simulink model "three_phase_inverter_reminder"  (R2020b)
settings: Solver=VariableStepAuto  StartTime=0.0  StopTime=0.3  RelTol=1e-3
InitFcn:
  | Tsys = 2e-6;
  | Udc = 380;
  | Tpwm = 1e-4;
  | 
  | Rload = 5
  | Lload = 5e-3
libraries: powerlib x25, simulink x1
settings Model: Creator=messer  LastModifiedBy=messer

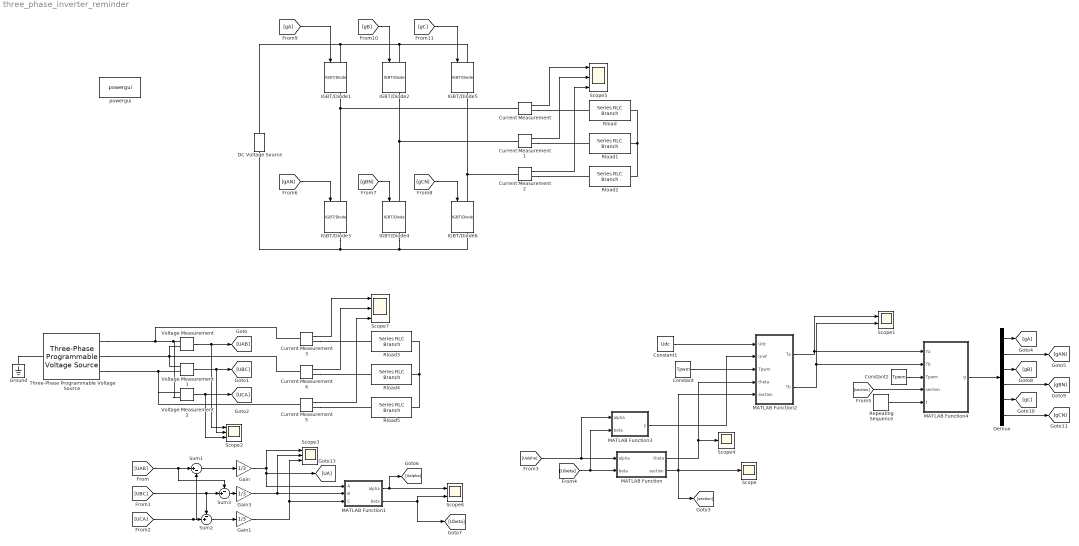
== system three_phase_inverter_reminder ==
  Constant : Constant  Value=Tpwm
  Constant1 : Constant  Value=Udc
  Constant2 : Constant  Value=Tpwm
  Current Measurement{,1..5} (6 alike) : powerlib/Measurements/Current Measurement  PhasorSimulation=off  OutputType=Complex  PSBequivalent=0
  DC Voltage Source : powerlib/Electrical Sources/DC Voltage Source  Amplitude=Udc  Measurements=None
  Demux : Demux  Outputs=6
  Gain : Gain  Gain=1/3
  Gain1 : Gain  Gain=1/3
  Gain3 : Gain  Gain=1/3
  Ground : powerlib/Elements/Ground  LConnTagsString=a
  IGBT/Diode{1..6} (6 alike) : powerlib/Power Electronics/IGBT//Diode  Ron=1e-3  Rs=1e5  Cs=inf  Measurements=on
  MATLAB Function : MATLAB Function  TreatAsAtomicUnit=on
  MATLAB Function1 : MATLAB Function  TreatAsAtomicUnit=on
  MATLAB Function2 : MATLAB Function  TreatAsAtomicUnit=on
  MATLAB Function3 : MATLAB Function  TreatAsAtomicUnit=on
  MATLAB Function4 : MATLAB Function  TreatAsAtomicUnit=on
  Repeating Sequence : simulink/Sources/Repeating Sequence  rep_seq_t=[0 Tpwm]  rep_seq_y=[0 Tpwm]
  Rload{,1..5} (6 alike) : powerlib/Elements/Series RLC Branch  LConnTagsString=__new0  RConnTagsString=__new0  BranchType=RL  Resistance=Rload  Inductance=Lload  SetiL0=off  InitialCurrent=0  Capacitance=1e-6  Setx0=off  InitialVoltage=0  Measurements=None
  Scope : Scope
  Scope1 : Scope  NumInputPorts=2
  Scope{2..3,5,7} (4 alike) : Scope  NumInputPorts=3
  Scope4 : Scope
  Scope6 : Scope  NumInputPorts=2
  Sum1 : Sum  Inputs=|+-
  Sum2 : Sum  Inputs=-+|
  Sum3 : Sum  Inputs=-+|
  Three-Phase Programmable Voltage Source : powerlib/Electrical Sources/Three-Phase Programmable Voltage Source  PositiveSequence="[380/sqrt(2)  0 50]"  VariationEntity=None  VariationType=Table of time-amplitude pairs  VariationTypeAlt=Step  VariationStep=0.5  VariationRate=10  VariationMagnitude=0.3  VariationFrequency=2  VariationTiming=[1 2]  VariationPhaseA=off  Amplitudes=[1 0.8 1.2 1.0]  TimeValues=[0 0.1 0.15 0.2]  HarmonicGeneration=off  HarmonicA=[3 0.2 -25 0]  HarmonicB=[2 0.15 35 2]  Timing="[0.05  3]"  BusType=swing  Pref=0  Qref=0  Qmin=-inf  Qmax=inf
  Voltage Measurement : powerlib/Measurements/Voltage Measurement  PhasorSimulation=off  OutputType=Complex  PSBequivalent=0
  Voltage Measurement1 : powerlib/Measurements/Voltage Measurement  PhasorSimulation=off  OutputType=Complex  PSBequivalent=0
  Voltage Measurement2 : powerlib/Measurements/Voltage Measurement  PhasorSimulation=off  OutputType=Complex  PSBequivalent=0
  powergui : powerlib/powergui  Priority=1  SimulationMode=Discrete  SampleTime=Tsys  frequency=60  Iterations=50  frequencyindice=50  Pbase=100e6  ErrMax=1e-4  UnitsV=kV  UnitsW=MW  buscounter=0  FunctionMessages=off  echomessages=off  EnableUseOfTLC=off  CurrentSourceSwitches=off  DisableSnubberDevices=off  DisableRonSwitches=off  DisableVfSwitches=off  DisplayEquations=off  AutomaticDiscreteSolvers=off  SolverType=Tustin/Backward Euler (TBE)  Interpol=off  ExternalGateDelay=off  methode=off  Ts=100  x0status=blocks  SPID=on  SwTol=0  HookPort=off  NonlinearTolerance=1e-4  nMaxIteration=100  ContinueOnMaxIteration=off  RestoreLinks=warning  ResistiveCurrentMeasurement=off  Frange=[0:2:500]  Ylog=off  Xlog=on  ShowGrid=off  save=off  variable=ZData  structure=0  ZoomFFT=off  StartTime=0.0  cycles=1  DisplayStyle=1  fundamental=60  FreqAxis=off  MaxFrequency=1000  frequencyindicesteady=1  RmsSteady=1  display=off
  wires:
  Voltage Measurement1/1 -> [UBC], Scope2/2
  Voltage Measurement2/1 -> [UCA], Scope2/3
  Voltage Measurement/1 -> Scope2/1, [UAB]
  Sum3/1 -> Gain3/1
  Sum1/1 -> Gain/1
  Gain3/1 -> MATLAB Function1/2(B), Scope3/2
  [UBC] -> Sum2/1, Sum3/2
  MATLAB Function1/1(alpha) -> [Ualpha], Scope6/1
  Gain/1 -> [UA], MATLAB Function1/1(A), Scope3/1
  Sum2/1 -> Gain1/1
  Gain1/1 -> MATLAB Function1/3(C), Scope3/3
  [UCA] -> Sum1/2, Sum2/2
  MATLAB Function1/2(beta) -> [Ubeta], Scope6/2
  [UAB] -> Sum3/1, Sum1/1
  [Ubeta] -> MATLAB Function3/2(beta), MATLAB Function/2(beta)
  MATLAB Function/2(section) -> [section], MATLAB Function2/5(section), Scope/1
  [Ualpha] -> MATLAB Function3/1(alpha), MATLAB Function/1(alpha)
  Constant/1 -> MATLAB Function2/3(Tpwm)
  MATLAB Function3/1(y) -> MATLAB Function2/2(Uref)
  Constant1/1 -> MATLAB Function2/1(Udc)
  MATLAB Function2/1(Ta) -> MATLAB Function4/1(Ta), Scope1/1
  MATLAB Function2/2(Tb) -> Scope1/2, MATLAB Function4/2(Tb)
  MATLAB Function/1(theta) -> MATLAB Function2/4(theta), Scope4/1
  Repeating Sequence/1 -> MATLAB Function4/5(t)
  [section] -> MATLAB Function4/4(section)
  Constant2/1 -> MATLAB Function4/3(Tpwm)
  Current Measurement/1 -> Scope5/1
  Current Measurement2/1 -> Scope5/3
  Current Measurement1/1 -> Scope5/2
  MATLAB Function4/1(g) -> Demux/1
  Demux/1 -> [gA]
  Demux/2 -> [gAN]
  Demux/3 -> [gB]
  Demux/4 -> [gBN]
  Demux/5 -> [gC]
  Demux/6 -> [gCN]
  [gA] -> IGBT/Diode1/1
  [gB] -> IGBT/Diode2/1
  [gC] -> IGBT/Diode5/1
  [gCN] -> IGBT/Diode6/1
  [gBN] -> IGBT/Diode4/1
  [gAN] -> IGBT/Diode3/1
  Current Measurement5/1 -> Scope7/3
  Current Measurement3/1 -> Scope7/1
  Current Measurement4/1 -> Scope7/2
  connections:
  IGBT/Diode1/RConn1 -- IGBT/Diode3/LConn1 -- Current Measurement/LConn1
  IGBT/Diode2/RConn1 -- Current Measurement1/LConn1 -- IGBT/Diode4/LConn1
  IGBT/Diode5/RConn1 -- IGBT/Diode6/LConn1 -- Current Measurement2/LConn1
  DC Voltage Source/RConn1 -- IGBT/Diode1/LConn1 -- IGBT/Diode2/LConn1 -- IGBT/Diode5/LConn1
  DC Voltage Source/LConn1 -- IGBT/Diode4/RConn1 -- IGBT/Diode6/RConn1 -- IGBT/Diode3/RConn1
  Rload2/RConn1 -- Rload/RConn1 -- Rload1/RConn1
  Three-Phase Programmable Voltage Source/RConn2 -- Voltage Measurement/LConn2 -- Current Measurement4/LConn1 -- Voltage Measurement1/LConn1
  Three-Phase Programmable Voltage Source/RConn3 -- Current Measurement5/LConn1 -- Voltage Measurement2/LConn1 -- Voltage Measurement1/LConn2
  Three-Phase Programmable Voltage Source/RConn1 -- Current Measurement3/LConn1 -- Voltage Measurement2/LConn2 -- Voltage Measurement/LConn1
  Ground/LConn1 -- Three-Phase Programmable Voltage Source/LConn1
  Current Measurement/RConn1 -- Rload/LConn1
  Current Measurement1/RConn1 -- Rload1/LConn1
  Current Measurement2/RConn1 -- Rload2/LConn1
  Rload5/RConn1 -- Rload3/RConn1 -- Rload4/RConn1
  Current Measurement5/RConn1 -- Rload5/LConn1
  Current Measurement4/RConn1 -- Rload4/LConn1
  Current Measurement3/RConn1 -- Rload3/LConn1

== matlab function three_phase_inverter_reminder/MATLAB Function1 ==
  data: A input; alpha output; B input; C input; beta output
function [alpha, beta] = fcn(A, B, C)
k = 2/ 3;
alpha = k * (A - 0.5*B - 0.5*C);
beta = k * sqrt(3) / 2 * (B - C);

== matlab function three_phase_inverter_reminder/MATLAB Function ==
  data: theta output; alpha input; section output; beta input
function [theta, section] = fcn(alpha, beta)

if(beta >=0)
    if(alpha == 0)
        theta = pi/2;
    elseif(alpha >0)
        theta = atan(beta/alpha);
    else
        theta = pi + atan(beta/alpha);
    end
else
    if(alpha == 0)
        theta = 1.5*pi;
    elseif(alpha > 0)
        theta = 2*pi + atan(beta/alpha);
    else
        theta = pi + atan(beta/alpha);
    end
end


k = sqrt(3);
if(beta > 0)
    if(beta < alpha*k)
        section = 0;
    elseif(beta <= -alpha*k)
        section = 2;
    else
        section = 1;
    end
    
else
    if(beta >= -alpha*k)
        section = 5;
    elseif(beta > alpha*k)
        section = 3;
    else
        section = 4;
    end
end

== matlab function three_phase_inverter_reminder/MATLAB Function2 ==
  data: Udc input; Ta output; Uref input; Tpwm input; theta input; section input; Tb output
function [Ta, Tb] = fcn(Udc, Uref, Tpwm, theta, section)

theta = theta - section*pi/3;

Ta = sqrt(3)*Uref/Udc*sin(pi/3 - theta) * Tpwm;
Tb = sqrt(3)*Uref/Udc * sin(theta) * Tpwm;

== matlab function three_phase_inverter_reminder/MATLAB Function3 ==
  data: alpha input; y output; beta input
function y = fcn(alpha, beta)

y = sqrt(alpha*alpha + beta*beta);

== matlab function three_phase_inverter_reminder/MATLAB Function4 ==
  data: Ta input; g output; Tb input; Tpwm input; section input; t input
function g  = fcn(Ta, Tb, Tpwm, section, t)

gA = 0;
gB = 0;
gC = 0;

T0 = Tpwm - Ta - Tb;

% 七段式 SPWM，扇区 0~5，对应6个扇区

if(mod(section, 2) == 0 ) % 0、2、4扇区
    t1 = T0/4;
    t2 = t1 + Ta / 2;
    t3 = t2 + Tb / 2;
    t4 = t3 + T0 / 2;
    t5 = t4 + Tb / 2;
    t6 = t5 + Ta / 2;
    
    if(section == 0)
        gA = (t >=t1 && t <=t6);
        gB = (t >=t2 && t <= t5);
        gC = (t >=t3 && t <= t4);
    elseif(section == 2)
        gB = (t >=t1 && t <=t6);
        gC = (t >=t2 && t <= t5);
        gA = (t >=t3 && t <= t4);
    else
        gC = (t >=t1 && t <=t6);
        gA = (t >=t2 && t <= t5);
        gB = (t >=t3 && t <= t4);
    end
else
    t1 = T0/4;
    t2 = t1 + Tb / 2;
    t3 = t2 + Ta / 2;
    t4 = t3 + T0 / 2;
    t5 = t4 + Ta / 2;
    t6 = t5 + Tb / 2;
    
    if(section == 1)
        gB = (t >=t1 && t <=t6);
        gA = (t >=t2 && t <= t5);
        gC = (t >=t3 && t <= t4);
    elseif(section == 3)
        gC = (t >=t1 && t <=t6);
        gB = (t >=t2 && t <= t5);
        gA = (t >=t3 && t <= t4);
    else
        gA = (t >=t1 && t <=t6);
        gC = (t >=t2 && t <= t5);
        gB = (t >=t3 && t <= t4);        
    end
    
end


g = [gA, 1-gA, gB, 1-gB, gC, 1-gC];
